simulink model "Lab2_sim"  (R2024b)
settings: Solver=FixedStepAuto  StartTime=0.0  StopTime=100  FixedStep=1e-5  RelTol=1e-3
values from neighbouring files (symbols this model uses):
  b = 5    [Lab2.m]
  g = 9.80665    [Lab2.m]
  k = 6    [Lab2.m]
  l = 0.1    [Lab2.m]
  m = 2    [Lab2.m]
  v0 = 0    [Lab2.m]
  w = 0.5    [Lab2.m]
  x0 = 1    [Lab2.m]
settings Model: Creator=alejandromunozvazquez  LastModifiedBy=alejandromunozvazquez

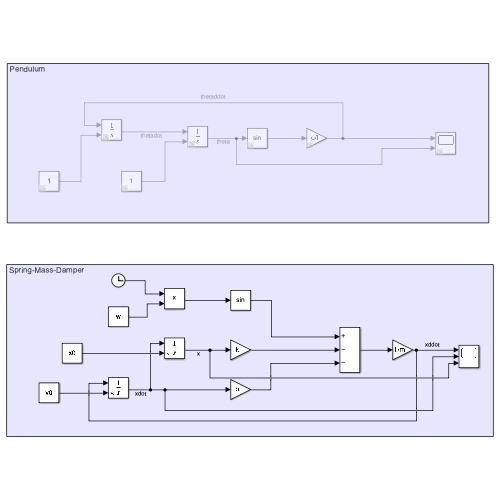
[thumbnail: Simulink's stored preview of the top-level diagram]
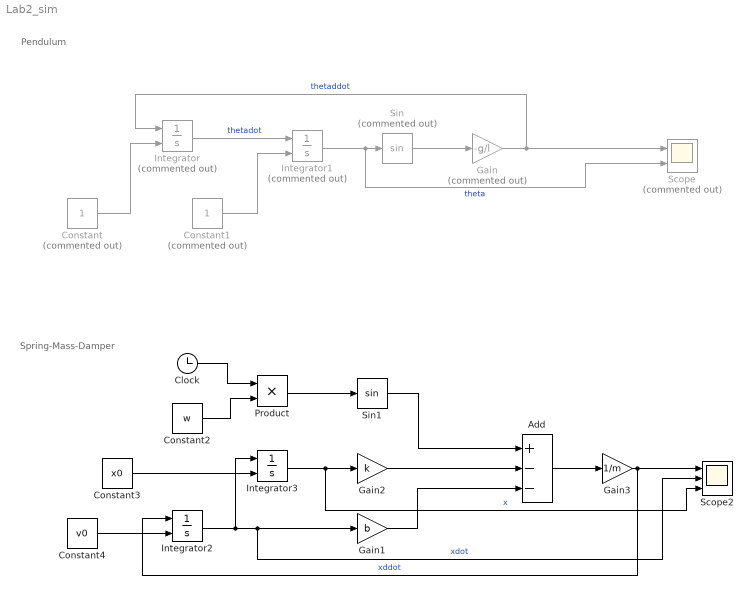
== system Lab2_sim ==
  note: Spring-Mass-Damper
  note: Pendulum
  Add : Sum  Inputs=+--
  Clock : Clock
  Constant : Constant  Commented=on
  Constant1 : Constant  Commented=on
  Constant2 : Constant  Value=w
  Constant3 : Constant  Value=x0
  Constant4 : Constant  Value=v0
  Gain : Gain  Commented=on  Gain=-g/l
  Gain1 : Gain  Gain=b
  Gain2 : Gain  Gain=k
  Gain3 : Gain  Gain=1/m
  Integrator : Integrator  Commented=on  InitialConditionSource=external
  Integrator1 : Integrator  Commented=on  InitialConditionSource=external
  Integrator2 : Integrator  InitialConditionSource=external
  Integrator3 : Integrator  InitialConditionSource=external
  Product : Product
  Scope : Scope  Commented=on  NumInputPorts=2
  Scope2 : Scope  NumInputPorts=3
  Sin : Trigonometry  Commented=on
  Sin1 : Trigonometry
  wires:
  Integrator/1 -> Integrator1/1  "thetadot"
  Sin/1 -> Gain/1
  Integrator1/1 -> Scope/2, Sin/1  "theta"
  Gain/1 -> Integrator/1, Scope/1  "thetaddot"
  Constant/1 -> Integrator/2
  Constant1/1 -> Integrator1/2
  Integrator2/1 -> Integrator3/1, Scope2/2, Gain1/1  "xdot"
  Integrator3/1 -> Scope2/3, Gain2/1  "x"
  Product/1 -> Sin1/1
  Clock/1 -> Product/1
  Constant2/1 -> Product/2
  Sin1/1 -> Add/1
  Gain3/1 -> Scope2/1, Integrator2/1  "xddot"
  Add/1 -> Gain3/1
  Gain2/1 -> Add/2
  Gain1/1 -> Add/3
  Constant3/1 -> Integrator3/2
  Constant4/1 -> Integrator2/2
